simulink model "SIGAS_Telemetry"  (R2026a)
settings: Solver=FixedStepDiscrete  StopTime=20  FixedStep=0.05
settings Model: Creator=josue  LastModifiedBy=josue

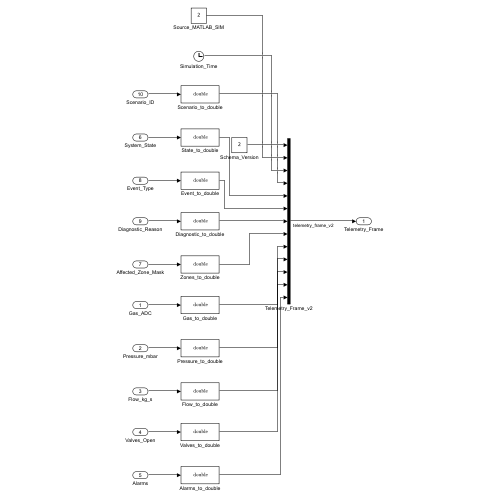
[thumbnail: Simulink's stored preview of the top-level diagram]
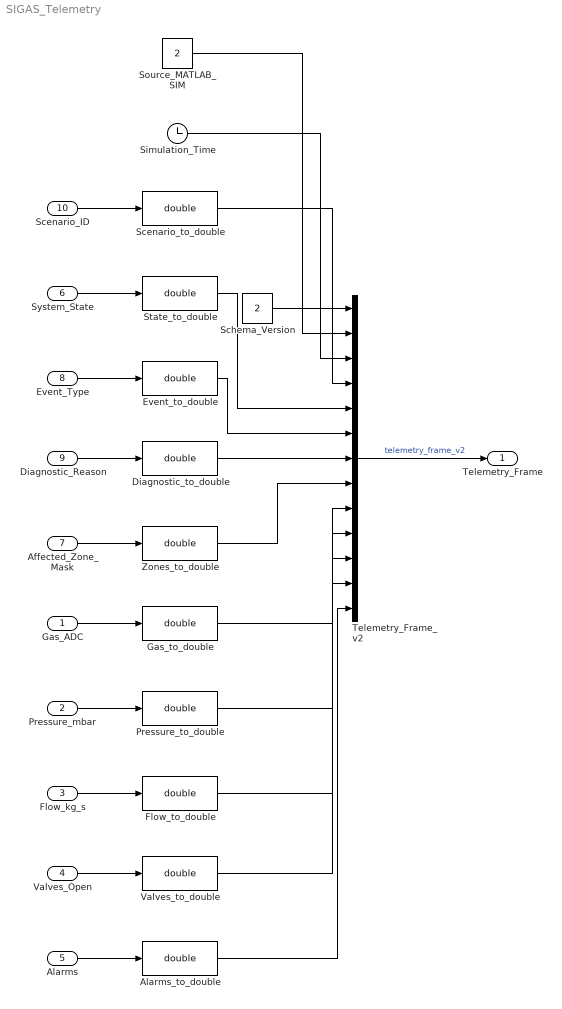
== system SIGAS_Telemetry ==
  Gas_ADC : Inport  OutDataTypeStr=uint16  PortDimensions=3
  Pressure_mbar : Inport  Port=2  OutDataTypeStr=double  PortDimensions=5
  Flow_kg_s : Inport  Port=3  OutDataTypeStr=double  PortDimensions=2
  Valves_Open : Inport  Port=4  OutDataTypeStr=boolean  PortDimensions=4
  Alarms : Inport  Port=5  OutDataTypeStr=boolean  PortDimensions=3
  System_State : Inport  Port=6  OutDataTypeStr=uint8  PortDimensions=1
  Affected_Zone_Mask : Inport  Port=7  OutDataTypeStr=uint8  PortDimensions=1
  Event_Type : Inport  Port=8  OutDataTypeStr=uint8  PortDimensions=1
  Diagnostic_Reason : Inport  Port=9  OutDataTypeStr=uint8  PortDimensions=1
  Scenario_ID : Inport  Port=10  OutDataTypeStr=double  PortDimensions=1
  Alarms_to_double : DataTypeConversion  OutDataTypeStr=double  SaturateOnIntegerOverflow=off  RndMeth=Floor
  Diagnostic_to_double : DataTypeConversion  OutDataTypeStr=double  SaturateOnIntegerOverflow=off  RndMeth=Floor
  Event_to_double : DataTypeConversion  OutDataTypeStr=double  SaturateOnIntegerOverflow=off  RndMeth=Floor
  Flow_to_double : DataTypeConversion  OutDataTypeStr=double  SaturateOnIntegerOverflow=off  RndMeth=Floor
  Gas_to_double : DataTypeConversion  OutDataTypeStr=double  SaturateOnIntegerOverflow=off  RndMeth=Floor
  Pressure_to_double : DataTypeConversion  OutDataTypeStr=double  SaturateOnIntegerOverflow=off  RndMeth=Floor
  Scenario_to_double : DataTypeConversion  OutDataTypeStr=double  SaturateOnIntegerOverflow=off  RndMeth=Floor
  Schema_Version : Constant  Value=2  OutDataTypeStr=double
  Simulation_Time : Clock
  Source_MATLAB_SIM : Constant  Value=2  OutDataTypeStr=double
  State_to_double : DataTypeConversion  OutDataTypeStr=double  SaturateOnIntegerOverflow=off  RndMeth=Floor
  Telemetry_Frame_v2 : Mux  Inputs=13
  Valves_to_double : DataTypeConversion  OutDataTypeStr=double  SaturateOnIntegerOverflow=off  RndMeth=Floor
  Zones_to_double : DataTypeConversion  OutDataTypeStr=double  SaturateOnIntegerOverflow=off  RndMeth=Floor
  Telemetry_Frame : Outport
  wires:
  Telemetry_Frame_v2/1 -> Telemetry_Frame/1  "telemetry_frame_v2"
  Simulation_Time/1 -> Telemetry_Frame_v2/3
  Source_MATLAB_SIM/1 -> Telemetry_Frame_v2/2
  Schema_Version/1 -> Telemetry_Frame_v2/1
  Gas_ADC/1 -> Gas_to_double/1
  Gas_to_double/1 -> Telemetry_Frame_v2/9
  Pressure_mbar/1 -> Pressure_to_double/1
  Pressure_to_double/1 -> Telemetry_Frame_v2/10
  Flow_kg_s/1 -> Flow_to_double/1
  Flow_to_double/1 -> Telemetry_Frame_v2/11
  Valves_Open/1 -> Valves_to_double/1
  Valves_to_double/1 -> Telemetry_Frame_v2/12
  Alarms/1 -> Alarms_to_double/1
  Alarms_to_double/1 -> Telemetry_Frame_v2/13
  System_State/1 -> State_to_double/1
  State_to_double/1 -> Telemetry_Frame_v2/5
  Affected_Zone_Mask/1 -> Zones_to_double/1
  Zones_to_double/1 -> Telemetry_Frame_v2/8
  Event_Type/1 -> Event_to_double/1
  Event_to_double/1 -> Telemetry_Frame_v2/6
  Diagnostic_Reason/1 -> Diagnostic_to_double/1
  Diagnostic_to_double/1 -> Telemetry_Frame_v2/7
  Scenario_ID/1 -> Scenario_to_double/1
  Scenario_to_double/1 -> Telemetry_Frame_v2/4
